simulink model "threeQ_cascaded_relays_R2024a"  (R2024a)
settings: Solver=VariableStepAuto  StartTime=0.0  StopTime=20  RelTol=1e-3
libraries: spsThreePhaseSeriesRLCLoadLib x2, spsThreePhaseVIMeasurementLib x2, spsThreePhaseBreakerLib x2, spsThreePhaseFaultLib x2, spsDistributedParametersLineLib x1, spsThreePhaseSourceLib x1, sps_lib x1
settings Model: SimulationMode=accelerator  Creator=Carnival  LastModifiedBy=Carnival

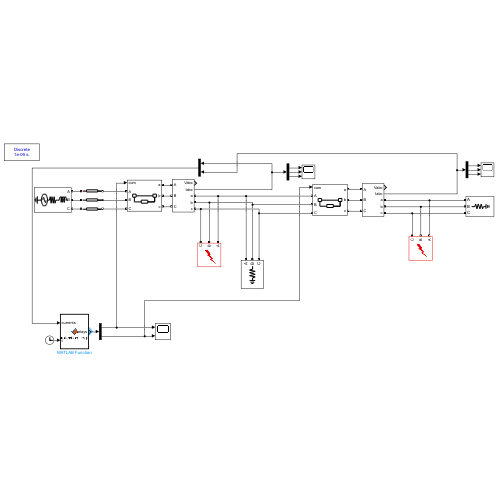
[thumbnail: Simulink's stored preview of the top-level diagram]
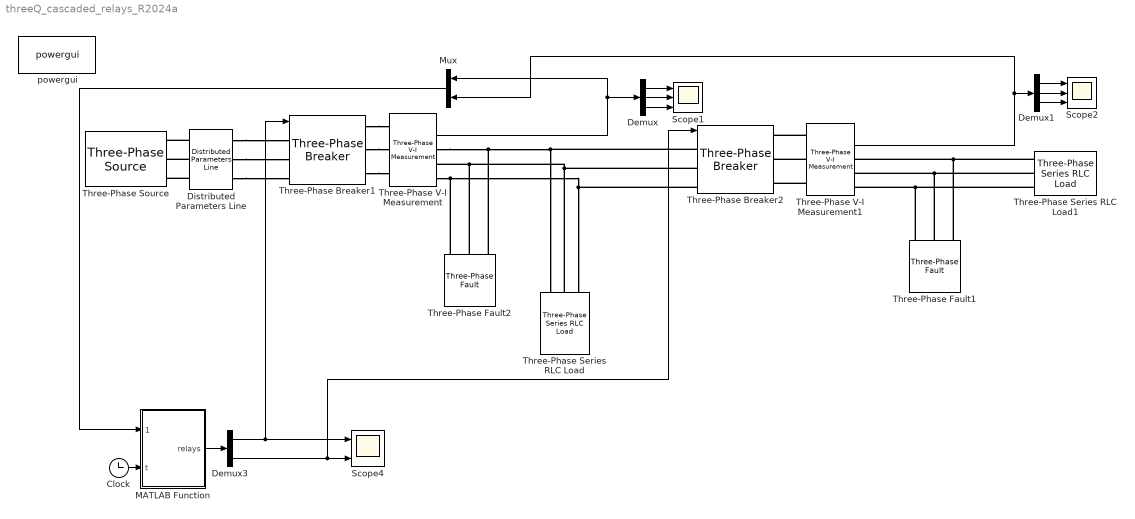
== system threeQ_cascaded_relays_R2024a ==
  Clock : Clock
  Demux : Demux  Outputs=3
  Demux1 : Demux  Outputs=3
  Demux3 : Demux  Outputs=2
  Distributed Parameters Line : spsDistributedParametersLineLib/Distributed Parameters Line  Phases=3  Length=100  Frequency=50  Resistance=[0.6273 0.8864]  Inductance="[0.9337e-3  4.1264e-3]"  Capacitance=[12.74e-9 7.751e-9]  x1=[-0.00057 2.24147551584483e-14 0 0;-0.00056 2.24642541014745e-14 0 0;-0.00055 2.25135313313819e-14 0 0;-0.00054 2.25625863618241e-14 0 0;-0.00053 2.26114187086478e-14 0 0;-0.00052 2.26600278898975e-14 0 0;-0.00051 2.27084134258201e-14 0 0;-0.0005 2.27565748388699e-14 0 0;-0.00049 2.28045116537133e-14 0 0;-0.00048 2.28522233972332e-14 0 0;-0.00047 2.28997095985341e-14 0 0;-0.00046 2.29469697889461e-14 0 0;-0.00045 2.29940035020304e-14 0 0;-0.00044 2.30408102735832e-14 0 0;-0.00043 2.30873896416406e-14 0 0;-0.00042 2.31337411464829e-14 0 0;-0.00041 2.31798643306396e-14 0 0;-0.0004 2.32257587388935e-14 0 0;-0.00039 2.32714239182852e-14 0 0;-0.00038 2.33168594181179e-14 0 0;-0.00037 2.33620647899615e-14 0 0;-0.00036 2.34070395876573e-14 0 0;-0.00035 2.34517833673222e-14 10.6712382260612 -27.4117386699955;-0.00034 2.34962956873531e-14 10.7573019408265 -27.3780787701286;-0.00033 2.35405761084314e-14 10.8432594853645 -27.3441486596772;-0.00032 2.35846241935272e-14 10.9291100113091 -27.3099486735179;-0.00031 2.36284395079038e-14 11.01485267135 -27.2754791491906;-0.0003 2.36720216191216e-14 11.100486619242 -27.2407404268956;-0.00029 2.37153700970428e-14 11.1860110098125 -27.2057328494902;-0.00028 2.37584845138354e-14 11.2714249989703 -27.1704567624849;-0.00027 2.38013644439775e-14 11.3567277437138 -27.1349125140406;-0.00026 2.38440094642616e-14 11.4419184021394 -27.0991004549646;-0.00025 2.38864191537985e-14 11.5269961334496 -27.0630209387074;-0.00024 2.39285930940217e-14 11.6119600979616 -27.0266743213593;-0.00023 2.39705308686914e-14 11.6968094571155 -26.9900609616468;-0.00022 2.40122320638987e-14 11.7815433734821 -26.9531812209289;-0.00021 2.40536962680697e-14 11.8661610107721 -26.9160354631938;-0.0002 2.40949230719694e-14 11.9506615338434 -26.8786240550552;-0.00019 2.41359120687059e-14 12.0350441087101 -26.8409473657484;-0.00018 2.41766628537343e-14 12.1193079025502 -26.8030057671273;-0.00017 2.42171750248609e-14 12.2034520837141 -26.7647996336601;-0.00016 2.42574481822468e-14 12.2874758217326 -26.7263293424259;-0.00015 2.42974819284124e-14 12.3713782873254 -26.6875952731109;-0.00014 2.43372758682405e-14 12.455158652409 -26.6485978080048;-0.00013 2.43768296089812e-14 12.5388160901051 -26.6093373319968;-0.00012 2.4416142760255e-14 12.6223497747485 -26.5698142325719;-0.00011 2.4455214934057e-14 12.7057588818955 -26.5300288998073;-0.0001 2.44940457447605e-14 12.7890425883318 -26.489981726368;-9e-05 2.45326348091212e-14 12.872200072081 -26.4496731075035;-8e-05 2.45709817462805e-14 12.9552305124121 -26.4091034410436;-7e-05 2.46090861777697e-14 13.0381330898483 -26.3682731273946;-6e-05 2.46469477275134e-14 13.1209069861747 -26.327182569535;-5e-05 2.46845660218334e-14 13.2035513844462 -26.2858321730122;-4e-05 2.47219406894523e-14 13.286065468996 -26.2442223459379;-3e-05 2.47590713614973e-14 13.3684484254434 -26.2023534989843;-2e-05 2.47959576715036e-14 13.450699440702 -26.1602260453799;-1e-05 2.48325992554182e-14 13.5328177029873 -26.1178404009058]  x2=[-0.00057 -1.83093755768515e-15 0 0;-0.00056 -1.84614786454705e-15 0 0;-0.00055 -1.86133995067486e-15 0 0;-0.00054 -1.8765136661288e-15 0 0;-0.00053 -1.89166886115044e-15 0 0;-0.00052 -1.90680538616411e-15 0 0;-0.00051 -1.92192309177843e-15 0 0;-0.0005 -1.93702182878775e-15 0 0;-0.00049 -1.95210144817363e-15 0 0;-0.00048 -1.9671618011063e-15 0 0;-0.00047 -1.98220273894618e-15 0 0;-0.00046 -1.99722411324527e-15 0 0;-0.00045 -2.01222577574867e-15 0 0;-0.00044 -2.02720757839604e-15 0 0;-0.00043 -2.04216937332302e-15 0 0;-0.00042 -2.05711101286275e-15 0 0;-0.00041 -2.07203234954727e-15 0 0;-0.0004 -2.08693323610901e-15 0 0;-0.00039 -2.10181352548224e-15 0 0;-0.00038 -2.11667307080451e-15 0 0;-0.00037 -2.13151172541811e-15 0 0;-0.00036 -2.1463293428715e-15 0 0;-0.00035 -2.16112577692079e-15 1.15392666499314 -11.8336136123279;-0.00034 -2.17590088153114e-15 1.1910973030352 -11.8299300542631;-0.00033 -2.19065451087824e-15 1.22825618542775 -11.8261297395645;-0.00032 -2.20538651934972e-15 1.26540294542761 -11.8222127057399;-0.00031 -2.2200967615466e-15 1.30253721641126 -11.8181789914486;-0.0003 -2.23478509228474e-15 1.33965863187845 -11.8140286365019;-0.00029 -2.24945136659623e-15 1.37676682545578 -11.8097616818621;-0.00028 -2.26409543973087e-15 1.41386143090036 -11.8053781696423;-0.00027 -2.27871716715758e-15 1.45094208210343 -11.8008781431059;-0.00026 -2.29331640456581e-15 1.48800841309391 -11.7962616466665;-0.00025 -2.30789300786696e-15 1.52506005804208 -11.791528725887;-0.00024 -2.32244683319587e-15 1.56209665126318 -11.7866794274794;-0.00023 -2.33697773691214e-15 1.59911782722097 -11.7817137993043;-0.00022 -2.35148557560163e-15 1.6361232205314 -11.7766318903705;-0.00021 -2.36597020607781e-15 1.67311246596617 -11.7714337508344;-0.0002 -2.38043148538325e-15 1.71008519845636 -11.7661194319994;-0.00019 -2.39486927079094e-15 1.74704105309603 -11.7606889863159;-0.00018 -2.40928341980578e-15 1.78397966514582 -11.75514246738;-0.00017 -2.42367379016593e-15 1.82090067003654 -11.7494799299337;-0.00016 -2.43804023984425e-15 1.85780370337277 -11.7437014298639;-0.00015 -2.45238262704967e-15 1.89468840093647 -11.7378070242022;-0.00014 -2.46670081022864e-15 1.93155439869057 -11.7317967711239;-0.00013 -2.48099464806646e-15 1.96840133278256 -11.7256707299478;-0.00012 -2.49526399948871e-15 2.00522883954807 -11.7194289611354;-0.00011 -2.50950872366267e-15 2.04203655551448 -11.7130715262905;-0.0001 -2.52372867999866e-15 2.07882411740448 -11.7065984881584;-9e-05 -2.53792372815145e-15 2.11559116213971 -11.7000099106253;-8e-05 -2.55209372802164e-15 2.15233732684426 -11.6933058587179;-7e-05 -2.56623853975706e-15 2.18906224884833 -11.6864863986025;-6e-05 -2.58035802375412e-15 2.22576556569176 -11.6795515975843;-5e-05 -2.59445204065923e-15 2.26244691512764 -11.6725015241071;-4e-05 -2.60852045137011e-15 2.29910593512585 -11.6653362477523;-3e-05 -2.62256311703724e-15 2.33574226387667 -11.6580558392381;-2e-05 -2.63657989906518e-15 2.37235553979432 -11.6506603704194;-1e-05 -2.65057065911394e-15 2.40894540152056 -11.6431499142864]  x3=[-0.00057 3.2420376948028e-17 0 0;-0.00056 3.18575319286643e-17 0 0;-0.00055 3.12943724883218e-17 0 0;-0.00054 3.0730904185157e-17 0 0;-0.00053 3.01671325803744e-17 0 0;-0.00052 2.96030632381723e-17 0 0;-0.00051 2.90387017256872e-17 0 0;-0.0005 2.84740536129394e-17 0 0;-0.00049 2.7909124472778e-17 0 0;-0.00048 2.73439198808254e-17 0 0;-0.00047 2.67784454154227e-17 0 0;-0.00046 2.62127066575747e-17 0 0;-0.00045 2.56467091908944e-17 0 0;-0.00044 2.50804586015485e-17 0 0;-0.00043 2.45139604782015e-17 0 0;-0.00042 2.39472204119613e-17 0 0;-0.00041 2.33802439963236e-17 0 0;-0.0004 2.28130368271165e-17 0 0;-0.00039 2.2245604502446e-17 0 0;-0.00038 2.167795262264e-17 0 0;-0.00037 2.11100867901933e-17 0 0;-0.00036 2.05420126097125e-17 0 0;-0.00035 1.99737356878603e-17 0.00334188793136192 0.146809920564145;-0.00034 1.94052616333007e-17 0.00288065523057227 0.146819694920126;-0.00033 1.88365960566429e-17 0.00241939409887847 0.146828020224992;-0.00032 1.82677445703867e-17 0.00195810908874166 0.146834896396575;-0.00031 1.76987127888666e-17 0.00149680475285867 0.14684032336701;-0.0003 1.71295063281966e-17 0.00103548564411705 0.146844301082736;-0.00029 1.65601308062145e-17 0.000574156315550162 0.146846829504493;-0.00028 1.5990591842427e-17 0.000112821320292235 0.146847908607328;-0.00027 1.54208950579536e-17 -0.000348514788466569 0.146847538380589;-0.00026 1.48510460754717e-17 -0.000809847457525118 0.146845718827931;-0.00025 1.42810505191606e-17 -0.0012711721337162 0.146842449967313;-0.00024 1.37109140146464e-17 -0.00173248426395153 0.146837731830996;-0.00023 1.31406421889462e-17 -0.0021937792952666 0.146831564465547;-0.00022 1.25702406704127e-17 -0.00265505267486569 0.146823947931835;-0.00021 1.19997150886786e-17 -0.00311629985016677 0.146814882305031;-0.0002 1.1429071074601e-17 -0.00357751626884642 0.146804367674611;-0.00019 1.08583142602061e-17 -0.00403869737888481 0.14679240414435;-0.00018 1.0287450278633e-17 -0.00449983862861055 0.146778991832322;-0.00017 9.71648476407896e-18 -0.00496093546674569 0.146764130870902;-0.00016 9.14542335174296e-18 -0.00542198334245058 0.146747821406761;-0.00015 8.57427167777064e-18 -0.00588297770536882 0.146730063600867;-0.00014 8.00303537919844e-18 -0.00634391400567217 0.146710857628483;-0.00013 7.431720093898e-18 -0.00680478769410542 0.146690203679164;-0.00012 6.86033146052054e-18 -0.00726559422203134 0.146668101956755;-0.00011 6.28887511844119e-18 -0.00772632904147552 0.146644552679393;-0.0001 5.71735670770335e-18 -0.00818698760517131 0.146619556079498;-9e-05 5.14578186896299e-18 -0.00864756536660466 0.146593112403778;-8e-05 4.57415624343302e-18 -0.009108057780059 0.14656522191322;-7e-05 4.00248547282759e-18 -0.00956846030066012 0.146535884883093;-6e-05 3.43077519930641e-18 -0.010028768384421 0.146505101602941;-5e-05 2.85903106541907e-18 -0.0104889774882867 0.146472872376582;-4e-05 2.28725871404936e-18 -0.0109490830701792 0.146439197522107;-3e-05 1.71546378835954e-18 -0.0114090805890421 0.146404077371872;-2e-05 1.14365193173469e-18 -0.0118689655048857 0.146367512272499;-1e-05 5.71828787726983e-19 -0.0123287332788313 0.146329502584871]  x4=[-0.00057 -6.40827426336711e-17 0 0;-0.00056 -6.34309035199778e-17 0 0;-0.00055 -6.27784383688748e-17 0 0;-0.00054 -6.21253536199298e-17 0 0;-0.00053 -6.14716557188256e-17 0 0;-0.00052 -6.08173511172966e-17 0 0;-0.00051 -6.0162446273065e-17 0 0;-0.0005 -5.95069476497772e-17 0 0;-0.00049 -5.88508617169401e-17 0 0;-0.00048 -5.81941949498568e-17 0 0;-0.00047 -5.75369538295634e-17 0 0;-0.00046 -5.68791448427643e-17 0 0;-0.00045 -5.62207744817686e-17 0 0;-0.00044 -5.5561849244426e-17 0 0;-0.00043 -5.49023756340626e-17 0 0;-0.00042 -5.42423601594167e-17 0 0;-0.00041 -5.35818093345745e-17 0 0;-0.0004 -5.29207296789061e-17 0 0;-0.00039 -5.22591277170007e-17 0 0;-0.00038 -5.15970099786025e-17 0 0;-0.00037 -5.09343829985465e-17 0 0;-0.00036 -5.02712533166933e-17 0 0;-0.00035 -4.96076274778652e-17 0.026418092350592 -0.270919727167897;-0.00034 -4.89435120317813e-17 0.0272690800071875 -0.270835395485401;-0.00033 -4.82789135329929e-17 0.0281197985289723 -0.270748390766893;-0.00032 -4.76138385408189e-17 0.0289702395196981 -0.270658713871073;-0.00031 -4.69482936192811e-17 0.0298203945858556 -0.270566365683017;-0.0003 -4.6282285337039e-17 0.0306702553367575 -0.270471347114163;-0.00029 -4.56158202673255e-17 0.0315198133846213 -0.270373659102307;-0.00028 -4.49489049878819e-17 0.032369060344652 -0.27027330261159;-0.00027 -4.42815460808926e-17 0.0332179878351251 -0.27017027863249;-0.00026 -4.36137501329207e-17 0.0340665874774689 -0.270064588181812;-0.00025 -4.29455237348426e-17 0.0349148508963475 -0.269956232302679;-0.00024 -4.2276873481783e-17 0.0357627697197434 -0.269845212064518;-0.00023 -4.160780597305e-17 0.0366103355790403 -0.269731528563055;-0.00022 -4.09383278120698e-17 0.0374575401091052 -0.2696151829203;-0.00021 -4.02684456063216e-17 0.0383043749483714 -0.269496176284538;-0.0002 -3.95981659672722e-17 0.0391508317389209 -0.269374509830315;-0.00019 -3.89274955103112e-17 0.0399969021265671 -0.269250184758432;-0.00018 -3.82564408546852e-17 0.0408425777609366 -0.269123202295926;-0.00017 -3.75850086234327e-17 0.0416878502955525 -0.268993563696062;-0.00016 -3.69132054433188e-17 0.042532711387916 -0.268861270238322;-0.00015 -3.62410379447696e-17 0.0433771526995893 -0.268726323228389;-0.00014 -3.5568512761807e-17 0.0442211658962775 -0.268588723998134;-0.00013 -3.4895636531983e-17 0.0450647426479111 -0.268448473905607;-0.00012 -3.42224158963144e-17 0.0459078746287281 -0.26830557433502;-0.00011 -3.3548857499217e-17 0.0467505535173564 -0.268160026696733;-0.0001 -3.28749679884403e-17 0.0475927709968953 -0.268011832427244;-9e-05 -3.22007540150018e-17 0.0484345187549985 -0.267860992989169;-8e-05 -3.15262222331211e-17 0.0492757884839554 -0.267707509871233;-7e-05 -3.08513793001546e-17 0.0501165718807734 -0.267551384588253;-6e-05 -3.01762318765296e-17 0.0509568606472598 -0.267392618681122;-5e-05 -2.95007866256786e-17 0.0517966464901038 -0.267231213716795;-4e-05 -2.88250502139736e-17 0.052635921120958 -0.267067171288274;-3e-05 -2.81490293106601e-17 0.0534746762565207 -0.266900493014592;-2e-05 -2.74727305877916e-17 0.0543129036186174 -0.266731180540796;-1e-05 -2.67961607201633e-17 0.0551505949342824 -0.266559235537932]  x5=0.000565541566995743  V1=ones(3,3)  V2=ones(3,3)  I1=ones(3,3)  I2=ones(3,3)  nHarmo=1  Measurements=None  Decoupling=off  VsMag0=0  VrMag0=0  VsAngle0=0  VrAngle0=0  IsMag0=0  IrMag0=0  IsAngle0=0  IrAngle0=0
      settings: LibrarySourceBlock=sps_lib/Power Grid Elements/Distributed Parameters Line
  MATLAB Function : MATLAB Function  TreatAsAtomicUnit=on
  Mux : Mux  Inputs=2
  Scope1 : Scope  NumInputPorts=3
  Scope2 : Scope  NumInputPorts=3
  Scope4 : Scope  NumInputPorts=2
  Three-Phase Series RLC Load : spsThreePhaseSeriesRLCLoadLib/Three-Phase Series RLC Load  LConnTagsString=A|B|C  Configuration=Y (grounded)  NominalVoltage=30  Vabc=[1e3 1e3 1e3]  Vabcp=[1e3 1e3 1e3]  NominalFrequency=50  UnbalancedPower=off  ActivePower=10  InductivePower=0  CapacitivePower=0  Pabc=[10e3 9e3 11e3]  QLabc=[100 90 110]  QCabc=[100 90 110]  Pabcp=[10e3 9e3 11e3]  QLabcp=[100 90 110]  QCabcp=[100 90 110]  Measurements=None  LoadType=constant Z
  Three-Phase Series RLC Load1 : spsThreePhaseSeriesRLCLoadLib/Three-Phase Series RLC Load  LConnTagsString=A|B|C  Configuration=Y (grounded)  NominalVoltage=30  Vabc=[1e3 1e3 1e3]  Vabcp=[1e3 1e3 1e3]  NominalFrequency=50  UnbalancedPower=off  ActivePower=10  InductivePower=0  CapacitivePower=0  Pabc=[10e3 9e3 11e3]  QLabc=[100 90 110]  QCabc=[100 90 110]  Pabcp=[10e3 9e3 11e3]  QLabcp=[100 90 110]  QCabcp=[100 90 110]  Measurements=None  LoadType=constant Z
  Three-Phase V-I Measurement : spsThreePhaseVIMeasurementLib/Three-Phase V-I Measurement  VoltageMeasurement=phase-to-ground  SetLabelV=off  LabelV=Vabc  Vpu=off  VpuLL=off  CurrentMeasurement=yes  SetLabelI=off  LabelI=Iabc  Ipu=off  Pbase=100e6  Vbase=500e3  OutputType=Complex  PhasorSimulation=off  PSBequivalent=0
  Three-Phase V-I Measurement1 : spsThreePhaseVIMeasurementLib/Three-Phase V-I Measurement  VoltageMeasurement=phase-to-ground  SetLabelV=off  LabelV=Vabc  Vpu=off  VpuLL=off  CurrentMeasurement=yes  SetLabelI=off  LabelI=Iabc  Ipu=off  Pbase=100e6  Vbase=500e3  OutputType=Complex  PhasorSimulation=off  PSBequivalent=0
  Three-Phase Breaker1 : spsThreePhaseBreakerLib/Three-Phase Breaker  InitialState=closed  SwitchA=on  SwitchB=on  SwitchC=on  SwitchTimes="[1/60  5/60]"  External=on  BreakerResistance=0.01  SnubberResistance=1e6  SnubberCapacitance=inf  Measurements=None
  Three-Phase Breaker2 : spsThreePhaseBreakerLib/Three-Phase Breaker  InitialState=closed  SwitchA=on  SwitchB=on  SwitchC=on  SwitchTimes="[1/60  5/60]"  External=on  BreakerResistance=0.01  SnubberResistance=1e6  SnubberCapacitance=inf  Measurements=None
  Three-Phase Fault1 : spsThreePhaseFaultLib/Three-Phase Fault  InitialStates=0  FaultA=on  FaultB=on  FaultC=on  GroundFault=on  SwitchTimes="[10  11]"  External=off  SwitchStatus=NaN  FaultResistance=0.001  GroundResistance=0.01  SnubberResistance=1e6  SnubberCapacitance=inf  Measurements=None
  Three-Phase Fault2 : spsThreePhaseFaultLib/Three-Phase Fault  InitialStates=0  FaultA=on  FaultB=on  FaultC=on  GroundFault=on  SwitchTimes="[5  6]"  External=off  SwitchStatus=NaN  FaultResistance=0.001  GroundResistance=0.01  SnubberResistance=1e6  SnubberCapacitance=inf  Measurements=None
  Three-Phase Source : spsThreePhaseSourceLib/Three-Phase Source  InternalConnection=Yg  VoltagePhases=off  Voltage=30  PhaseAngle=0  Voltage_phases=[25e3 25e3 25e3]/sqrt(3)  PhaseAngles_phases=[0 -120 +120]  Frequency=50  NonIdealSource=on  SpecifyImpedance=off  Resistance=0.8929  Inductance=16.58e-3  ShortCircuitLevel=100e6  BaseVoltage=30  XRratio=7  BusType=swing  Pref=10e3  Qref=0  Prefabc=[10e3, 10e3, 10e3]  Qrefabc=[0, 0, 0]  Qmin=-inf  Qmax=inf
  powergui : sps_lib/powergui  Priority=1  SimulationMode=Discrete  SampleTime=1e-5  frequency=60  Iterations=50  frequencyindice=0  Pbase=100e6  ErrMax=1e-4  UnitsV=kV  UnitsW=MW  buscounter=0  FunctionMessages=off  echomessages=off  EnableUseOfTLC=off  CurrentSourceSwitches=off  DisableSnubberDevices=off  DisableRonSwitches=off  DisableVfSwitches=off  DisplayEquations=off  AutomaticDiscreteSolvers=off  SolverType=Tustin/Backward Euler (TBE)  Interpol=off  ExternalGateDelay=off  methode=off  Ts=100  x0status=blocks  SPID=on  SwTol=0  HookPort=off  NonlinearTolerance=1e-4  nMaxIteration=100  ContinueOnMaxIteration=off  RestoreLinks=warning  ResistiveCurrentMeasurement=off  Frange=[0:2:500]  Ylog=off  Xlog=on  ShowGrid=off  save=off  variable=ZData  structure=0  ZoomFFT=off  StartTime=0.0  cycles=1  DisplayStyle=1  fundamental=60  FreqAxis=off  MaxFrequency=1000  frequencyindicesteady=1  RmsSteady=1  display=off
  wires:
  Three-Phase V-I Measurement/2 -> Mux/1, Demux/1
  Three-Phase V-I Measurement1/2 -> Demux1/1, Mux/2
  Demux/1 -> Scope1/1
  Demux/2 -> Scope1/2
  Demux/3 -> Scope1/3
  Demux1/1 -> Scope2/1
  Demux1/2 -> Scope2/2
  Demux1/3 -> Scope2/3
  Clock/1 -> MATLAB Function/2(t)
  Demux3/1 -> Scope4/1, Three-Phase Breaker1/1
  Demux3/2 -> Scope4/2, Three-Phase Breaker2/1
  Mux/1 -> MATLAB Function/1(currents)
  MATLAB Function/1(relays) -> Demux3/1
  connections:
  Three-Phase Breaker1/RConn1 -- Three-Phase V-I Measurement/LConn1
  Three-Phase Breaker1/RConn2 -- Three-Phase V-I Measurement/LConn2
  Three-Phase Breaker1/RConn3 -- Three-Phase V-I Measurement/LConn3
  Three-Phase V-I Measurement/RConn1 -- Three-Phase Breaker2/LConn1 -- Three-Phase Series RLC Load/LConn1 -- Three-Phase Fault2/LConn1
  Three-Phase Series RLC Load/LConn2 -- Three-Phase Fault2/LConn2 -- Three-Phase V-I Measurement/RConn2 -- Three-Phase Breaker2/LConn2
  Three-Phase V-I Measurement/RConn3 -- Three-Phase Breaker2/LConn3 -- Three-Phase Series RLC Load/LConn3 -- Three-Phase Fault2/LConn3
  Three-Phase V-I Measurement1/LConn1 -- Three-Phase Breaker2/RConn1
  Three-Phase V-I Measurement1/LConn2 -- Three-Phase Breaker2/RConn2
  Three-Phase V-I Measurement1/LConn3 -- Three-Phase Breaker2/RConn3
  Three-Phase Series RLC Load1/LConn3 -- Three-Phase Fault1/LConn3 -- Three-Phase V-I Measurement1/RConn3
  Three-Phase Series RLC Load1/LConn2 -- Three-Phase Fault1/LConn2 -- Three-Phase V-I Measurement1/RConn2
  Three-Phase Series RLC Load1/LConn1 -- Three-Phase Fault1/LConn1 -- Three-Phase V-I Measurement1/RConn1
  Distributed Parameters Line/LConn2 -- Three-Phase Source/RConn2
  Distributed Parameters Line/LConn3 -- Three-Phase Source/RConn3
  Distributed Parameters Line/LConn1 -- Three-Phase Source/RConn1
  Distributed Parameters Line/RConn1 -- Three-Phase Breaker1/LConn1
  Distributed Parameters Line/RConn2 -- Three-Phase Breaker1/LConn2
  Distributed Parameters Line/RConn3 -- Three-Phase Breaker1/LConn3

== matlab function threeQ_cascaded_relays_R2024a/MATLAB Function ==
  settings: updateMethod=DISCRETE
  data: currents input; relays output; t input
function relays = protection_logic(currents, t)

%% --- Persistent State ---
persistent load1_tripped load2_tripped
persistent tripTime1 tripTime2
persistent startFaultTime1 startFaultTime2
persistent timing1 timing2
persistent rms_buffer

if isempty(load1_tripped)
    load1_tripped   = false;
    load2_tripped   = false;
    tripTime1       = -inf;
    tripTime2       = -inf;
    startFaultTime1 = -inf;
    startFaultTime2 = -inf;
    timing1         = false;
    timing2         = false;
    rms_buffer      = zeros(50, 6);
end

%% --- Protection Settings ---
I_pickup = 0.22;
K        = 0.14;
alph     = 0.02;
TMS1     = 0.05;   % Upstream  — أبطأ
TMS2     = 0.01;   % Downstream — أسرع

%% --- Moving RMS ---
row        = reshape(currents, 1, 6);
rms_buffer = [rms_buffer(2:end, :); row];
rms_vals   = sqrt(mean(rms_buffer.^2, 1));

max1 = max(rms_vals(1:3));
max2 = max(rms_vals(4:6));

%% --- Trip Delay Inline ---
ratio2 = max2 / I_pickup;
if ratio2 > 1
    tripDelay2 = (K * TMS2) / (ratio2^alph - 1);
else
    tripDelay2 = inf;
end

ratio1 = max1 / I_pickup;
if ratio1 > 1
    tripDelay1 = (K * TMS1) / (ratio1^alph - 1);
else
    tripDelay1 = inf;
end

%% --- Downstream Protection (Load 2) ---
if max2 > I_pickup && ~load2_tripped
    if ~timing2
        startFaultTime2 = t;
        timing2         = true;
    end
    if (t - startFaultTime2) >= tripDelay2
        load2_tripped = true;
        tripTime2     = t;
        timing2       = false;
    end
else
    timing2 = false;
end

%% --- Upstream Protection (Load 1) ---
downstream_fault = (max2 > I_pickup) || load2_tripped;

if max1 > I_pickup && ~load1_tripped && ~downstream_fault
    if ~timing1
        startFaultTime1 = t;
        timing1         = true;
    end
    if (t - startFaultTime1) >= tripDelay1
        load1_tripped = true;
        tripTime1     = t;
        timing1       = false;
    end
else
    timing1 = false;
end

%% --- Auto-Reclose Load 2 ---
if load2_tripped && (t - tripTime2) > 1.0
    if max2 <= I_pickup
        load2_tripped = false;
    else
        tripTime2 = t;
    end
end

%% --- Auto-Reclose Load 1 ---
if load1_tripped && (t - tripTime1) > 1.0
    if max1 <= I_pickup
        load1_tripped = false;
    else
        tripTime1 = t;
    end
end

%% --- Output ---
r1 = double(~load1_tripped);
r2 = double(~load2_tripped);

relays = [r1; r2];
